simulink model "igct_diode"  (R2023b)
settings: Solver=VariableStepAuto  StartTime=0.0  StopTime=10.0  RelTol=1e-3
values from neighbouring files (symbols this model uses):
  temp_init = 40    [power_sysinit.m]
  Ts1 = 1e-6    (= 1e-06)    [power_sysinit.m]
  Ts2 = 500E-6    (= 0.0005)    [power_sysinit.m]
  Udc = 2500    [power_sysinit.m]
undefined symbols (not defined in the file or in its folder): DIODE_204520, DIODE_344520, DIODE_364520, DIODE_364521, DIODE_D1031SH, DIODE_D1331SH, IGCT_364520_36, IGCT_364521_36, IGCT_654522_6, magnitude, Rch_DIODE, Rch_tau_DIODE, Rjc1_DIODE, Rjc1_tau_DIODE, Rjc2_DIODE, Rjc2_tau_DIODE, Rjc3_DIODE, Rjc3_tau_DIODE, Rth_h, Rth_h_tau
libraries: spsMeanLib x304, simulink x52, spsRMSLib x52
(part 11 of 11)

== system igct_diode/IGCT/36L4521/Subsystem/Subsystem56 ==
  I : Inport
  pwm : Inport  Port=2
  Abs1 : Abs  SaturateOnIntegerOverflow=off
  Add : Sum
  Constant1 : Constant  Value=0
  Constant2 : Constant  Value=0
  Gain1 : Gain  Gain=Udc/IGCT_364521_36.Vdc
  Gain2 : Gain  Gain=IGCT_364521_36.Eon/IGCT_364521_36.IT*Udc/IGCT_364521_36.Vdc
  Gain3 : Gain  Gain=1/Ts2
  Gain4 : Gain
  Logical Operator : Logic  AllPortsSameDT=off  OutDataTypeStr=boolean
  Logical Operator1 : Logic  Operator=NOT  AllPortsSameDT=off  OutDataTypeStr=boolean
  Logical Operator2 : Logic  Operator=NOT  AllPortsSameDT=off  OutDataTypeStr=boolean
  Logical Operator3 : Logic  AllPortsSameDT=off  OutDataTypeStr=boolean
  Logical Operator4 : Logic  AllPortsSameDT=off  OutDataTypeStr=boolean
  Logical Operator5 : Logic  Operator=NOT  AllPortsSameDT=off  OutDataTypeStr=boolean
  Polynomial : Polyval  Coefs=IGCT_364521_36.poly
  Pulse Generator : DiscretePulseGenerator  PulseType=Time based  Period=Ts2  PulseWidth=5
  Switch{1..4} (4 alike) : Switch  Criteria=u2 > Threshold  SaturateOnIntegerOverflow=off  InputSameDT=off
  Unit Delay{,1..3} (4 alike) : UnitDelay  SampleTime=Ts1  HasFrameUpgradeWarning=on
  PS : Outport  VectorParamsAs1DForOutWhenUnconnected=off
  wires:
  pwm/1 -> Logical Operator2/1, Logical Operator/1, Unit Delay/1
  Logical Operator/1 -> Switch1/2
  Abs1/1 -> Add/1
  Switch1/1 -> Abs1/1
  Unit Delay/1 -> Logical Operator3/1, Logical Operator1/1
  Logical Operator1/1 -> Logical Operator/2
  Logical Operator2/1 -> Logical Operator3/2
  Logical Operator3/1 -> Switch2/2
  Constant2/1 -> Switch2/3
  Gain2/1 -> Switch1/1
  Gain1/1 -> Switch1/3
  Switch3/1 -> Add/2
  Constant1/1 -> Switch3/1
  Pulse Generator/1 -> Unit Delay3/1, Logical Operator4/1
  Switch4/1 -> Unit Delay2/1, Gain3/1
  Unit Delay2/1 -> Switch4/3
  Unit Delay3/1 -> Logical Operator5/1
  Logical Operator5/1 -> Logical Operator4/2
  Logical Operator4/1 -> Switch4/2, Switch3/2
  Unit Delay1/1 -> Switch3/3, Switch4/1
  Gain3/1 -> PS/1
  I/1 -> Gain4/1
  Add/1 -> Unit Delay1/1
  Gain4/1 -> Gain2/1, Polynomial/1
  Switch2/1 -> Gain1/1
  Polynomial/1 -> Switch2/1

== system igct_diode/IGCT/36L4521/Subsystem/导通损耗 ==
  note: IGCT导通损耗
  note: 1.39选用的是阈值电压、是否需要改为导通电压
  I : Inport
  Add : Sum
  Gain1 : Gain  Gain=IGCT_364521_36.rT
  Gain2 : Gain  Gain=IGCT_364521_36.VT0
  Gain3 : Gain
  Math Function : Math  Operator=magnitude^2  SignedPower=on
  PD : Outport  VectorParamsAs1DForOutWhenUnconnected=off
  wires:
  Add/1 -> PD/1
  Gain2/1 -> Add/2
  Math Function/1 -> Gain1/1
  I/1 -> Gain3/1
  Gain1/1 -> Add/1
  Gain3/1 -> Gain2/1, Math Function/1

== system igct_diode/IGCT/36L4521/Subsystem/导通损耗1 ==
  note: 1.39选用的是阈值电压、是否需要改为导通电压
  note: IGCT导通损耗
  I : Inport
  Add : Sum
  Gain1 : Gain  Gain=IGCT_364521_36.rT
  Gain2 : Gain  Gain=IGCT_364521_36.VT0
  Gain3 : Gain
  Math Function : Math  Operator=magnitude^2  SignedPower=on
  PD : Outport  VectorParamsAs1DForOutWhenUnconnected=off
  wires:
  Gain3/1 -> Math Function/1, Gain2/1
  Gain1/1 -> Add/1
  I/1 -> Gain3/1
  Math Function/1 -> Gain1/1
  Gain2/1 -> Add/2
  Add/1 -> PD/1

== system igct_diode/IGCT/65L4522/Subsystem/Subsystem1 ==
  I : Inport
  pwm : Inport  Port=2
  Abs1 : Abs  SaturateOnIntegerOverflow=off
  Add : Sum
  Constant1 : Constant  Value=0
  Constant2 : Constant  Value=0
  Gain1 : Gain  Gain=Udc/IGCT_654522_6.Vdc
  Gain2 : Gain  Gain=IGCT_654522_6.Eon/IGCT_654522_6.IT*Udc/IGCT_654522_6.Vdc
  Gain3 : Gain  Gain=1/Ts2
  Gain4 : Gain
  Logical Operator : Logic  AllPortsSameDT=off  OutDataTypeStr=boolean
  Logical Operator1 : Logic  Operator=NOT  AllPortsSameDT=off  OutDataTypeStr=boolean
  Logical Operator2 : Logic  Operator=NOT  AllPortsSameDT=off  OutDataTypeStr=boolean
  Logical Operator3 : Logic  AllPortsSameDT=off  OutDataTypeStr=boolean
  Logical Operator4 : Logic  AllPortsSameDT=off  OutDataTypeStr=boolean
  Logical Operator5 : Logic  Operator=NOT  AllPortsSameDT=off  OutDataTypeStr=boolean
  Polynomial : Polyval  Coefs=IGCT_654522_6.poly
  Pulse Generator : DiscretePulseGenerator  PulseType=Time based  Period=Ts2  PulseWidth=5
  Switch{1..4} (4 alike) : Switch  Criteria=u2 > Threshold  SaturateOnIntegerOverflow=off  InputSameDT=off
  Unit Delay{,1..3} (4 alike) : UnitDelay  SampleTime=Ts1  HasFrameUpgradeWarning=on
  PS : Outport  VectorParamsAs1DForOutWhenUnconnected=off
  wires:
  pwm/1 -> Logical Operator2/1, Logical Operator/1, Unit Delay/1
  Logical Operator/1 -> Switch1/2
  Abs1/1 -> Add/1
  Switch1/1 -> Abs1/1
  Unit Delay/1 -> Logical Operator3/1, Logical Operator1/1
  Logical Operator1/1 -> Logical Operator/2
  Logical Operator2/1 -> Logical Operator3/2
  Logical Operator3/1 -> Switch2/2
  Constant2/1 -> Switch2/3
  Gain2/1 -> Switch1/1
  Gain1/1 -> Switch1/3
  Switch3/1 -> Add/2
  Constant1/1 -> Switch3/1
  Pulse Generator/1 -> Unit Delay3/1, Logical Operator4/1
  Switch4/1 -> Unit Delay2/1, Gain3/1
  Unit Delay2/1 -> Switch4/3
  Unit Delay3/1 -> Logical Operator5/1
  Logical Operator5/1 -> Logical Operator4/2
  Logical Operator4/1 -> Switch4/2, Switch3/2
  Unit Delay1/1 -> Switch3/3, Switch4/1
  Gain3/1 -> PS/1
  I/1 -> Gain4/1
  Add/1 -> Unit Delay1/1
  Gain4/1 -> Gain2/1, Polynomial/1
  Switch2/1 -> Gain1/1
  Polynomial/1 -> Switch2/1

== system igct_diode/IGCT/65L4522/Subsystem/Subsystem2 ==
  note: ch_double
  AVG : Inport
  SW : Inport  Port=2
  Add1 : Sum  Inputs=5
  Add2 : Sum  Inputs=+++
  Add3 : Sum
  Constant1 : Constant  Value=temp_init
  Discrete Filter1 : DiscreteFilter  Numerator=[Ts2/IGCT_654522_6.Rth_ch_dou_tau]  Denominator=[1 (Ts2/IGCT_654522_6.Rth_ch_dou_tau)-1]  SampleTime=Ts2
  Discrete Filter2 : DiscreteFilter  Numerator=[Ts2/IGCT_654522_6.Rth_jc3_dou_tau]  Denominator=[1 (Ts2/IGCT_654522_6.Rth_jc3_dou_tau)-1]  SampleTime=Ts2
  Discrete Filter3 : DiscreteFilter  Numerator=[Ts2/IGCT_654522_6.Rth_jc4_dou_tau]  Denominator=[1 (Ts2/IGCT_654522_6.Rth_jc4_dou_tau)-1]  SampleTime=Ts2
  Discrete Filter5 : DiscreteFilter  Numerator=[Ts2/IGCT_654522_6.Rth_jc1_dou_tau]  Denominator=[1 (Ts2/IGCT_654522_6.Rth_jc1_dou_tau)-1]  SampleTime=Ts2
  Discrete Filter6 : DiscreteFilter  Numerator=[Ts2/IGCT_654522_6.Rth_jc2_dou_tau]  Denominator=[1 (Ts2/IGCT_654522_6.Rth_jc2_dou_tau)-1]  SampleTime=Ts2
  Discrete Filter9 : DiscreteFilter  Numerator=[Ts2/Rth_h_tau]  Denominator=[1 (Ts2/Rth_h_tau)-1]  SampleTime=Ts2
  Gain1 : Gain  Gain=IGCT_654522_6.Rth_ch_dou
  Gain5 : Gain  Gain=IGCT_654522_6.Rth_jc1_dou
  Gain6 : Gain  Gain=IGCT_654522_6.Rth_jc2_dou
  Gain7 : Gain  Gain=IGCT_654522_6.Rth_jc3_dou
  Gain8 : Gain  Gain=IGCT_654522_6.Rth_jc4_dou
  Gain9 : Gain  Gain=Rth_h
  TEMP : Outport  VectorParamsAs1DForOutWhenUnconnected=off
  wires:
  Add3/1 -> Gain9/1, Gain5/1, Gain6/1, Gain7/1, Gain8/1, Gain1/1
  Gain1/1 -> Discrete Filter1/1
  Discrete Filter1/1 -> Add1/5
  Add2/1 -> TEMP/1
  Add1/1 -> Add2/2
  Gain8/1 -> Discrete Filter3/1
  Discrete Filter5/1 -> Add1/1
  Discrete Filter3/1 -> Add1/4
  Discrete Filter2/1 -> Add1/3
  Constant1/1 -> Add2/3
  Gain7/1 -> Discrete Filter2/1
  Discrete Filter6/1 -> Add1/2
  Gain5/1 -> Discrete Filter5/1
  Discrete Filter9/1 -> Add2/1
  Gain9/1 -> Discrete Filter9/1
  Gain6/1 -> Discrete Filter6/1
  SW/1 -> Add3/2
  AVG/1 -> Add3/1

== system igct_diode/IGCT/65L4522/Subsystem/Subsystem31 ==
  note: ch_double
  AVG : Inport
  SW : Inport  Port=2
  Add1 : Sum  Inputs=5
  Add2 : Sum  Inputs=+++
  Add3 : Sum
  Constant1 : Constant  Value=temp_init
  Discrete Filter1 : DiscreteFilter  Numerator=[Ts2/IGCT_654522_6.Rth_ch_dou_tau]  Denominator=[1 (Ts2/IGCT_654522_6.Rth_ch_dou_tau)-1]  SampleTime=Ts2
  Discrete Filter2 : DiscreteFilter  Numerator=[Ts2/IGCT_654522_6.Rth_jc3_dou_tau]  Denominator=[1 (Ts2/IGCT_654522_6.Rth_jc3_dou_tau)-1]  SampleTime=Ts2
  Discrete Filter3 : DiscreteFilter  Numerator=[Ts2/IGCT_654522_6.Rth_jc4_dou_tau]  Denominator=[1 (Ts2/IGCT_654522_6.Rth_jc4_dou_tau)-1]  SampleTime=Ts2
  Discrete Filter5 : DiscreteFilter  Numerator=[Ts2/IGCT_654522_6.Rth_jc1_dou_tau]  Denominator=[1 (Ts2/IGCT_654522_6.Rth_jc1_dou_tau)-1]  SampleTime=Ts2
  Discrete Filter6 : DiscreteFilter  Numerator=[Ts2/IGCT_654522_6.Rth_jc2_dou_tau]  Denominator=[1 (Ts2/IGCT_654522_6.Rth_jc2_dou_tau)-1]  SampleTime=Ts2
  Discrete Filter9 : DiscreteFilter  Numerator=[Ts2/Rth_h_tau]  Denominator=[1 (Ts2/Rth_h_tau)-1]  SampleTime=Ts2
  Gain1 : Gain  Gain=IGCT_654522_6.Rth_ch_dou
  Gain5 : Gain  Gain=IGCT_654522_6.Rth_jc1_dou
  Gain6 : Gain  Gain=IGCT_654522_6.Rth_jc2_dou
  Gain7 : Gain  Gain=IGCT_654522_6.Rth_jc3_dou
  Gain8 : Gain  Gain=IGCT_654522_6.Rth_jc4_dou
  Gain9 : Gain  Gain=Rth_h
  TEMP : Outport  VectorParamsAs1DForOutWhenUnconnected=off
  wires:
  AVG/1 -> Add3/1
  SW/1 -> Add3/2
  Gain6/1 -> Discrete Filter6/1
  Gain9/1 -> Discrete Filter9/1
  Discrete Filter9/1 -> Add2/1
  Gain5/1 -> Discrete Filter5/1
  Discrete Filter6/1 -> Add1/2
  Gain7/1 -> Discrete Filter2/1
  Constant1/1 -> Add2/3
  Discrete Filter2/1 -> Add1/3
  Discrete Filter3/1 -> Add1/4
  Discrete Filter5/1 -> Add1/1
  Gain8/1 -> Discrete Filter3/1
  Add1/1 -> Add2/2
  Add2/1 -> TEMP/1
  Discrete Filter1/1 -> Add1/5
  Gain1/1 -> Discrete Filter1/1
  Add3/1 -> Gain1/1, Gain8/1, Gain7/1, Gain6/1, Gain5/1, Gain9/1

== system igct_diode/IGCT/65L4522/Subsystem/Subsystem56 ==
  I : Inport
  pwm : Inport  Port=2
  Abs1 : Abs  SaturateOnIntegerOverflow=off
  Add : Sum
  Constant1 : Constant  Value=0
  Constant2 : Constant  Value=0
  Gain1 : Gain  Gain=Udc/IGCT_654522_6.Vdc
  Gain2 : Gain  Gain=IGCT_654522_6.Eon/IGCT_654522_6.IT*Udc/IGCT_654522_6.Vdc
  Gain3 : Gain  Gain=1/Ts2
  Gain4 : Gain
  Logical Operator : Logic  AllPortsSameDT=off  OutDataTypeStr=boolean
  Logical Operator1 : Logic  Operator=NOT  AllPortsSameDT=off  OutDataTypeStr=boolean
  Logical Operator2 : Logic  Operator=NOT  AllPortsSameDT=off  OutDataTypeStr=boolean
  Logical Operator3 : Logic  AllPortsSameDT=off  OutDataTypeStr=boolean
  Logical Operator4 : Logic  AllPortsSameDT=off  OutDataTypeStr=boolean
  Logical Operator5 : Logic  Operator=NOT  AllPortsSameDT=off  OutDataTypeStr=boolean
  Polynomial : Polyval  Coefs=IGCT_654522_6.poly
  Pulse Generator : DiscretePulseGenerator  PulseType=Time based  Period=Ts2  PulseWidth=5
  Switch{1..4} (4 alike) : Switch  Criteria=u2 > Threshold  SaturateOnIntegerOverflow=off  InputSameDT=off
  Unit Delay{,1..3} (4 alike) : UnitDelay  SampleTime=Ts1  HasFrameUpgradeWarning=on
  PS : Outport  VectorParamsAs1DForOutWhenUnconnected=off
  wires:
  pwm/1 -> Logical Operator2/1, Logical Operator/1, Unit Delay/1
  Logical Operator/1 -> Switch1/2
  Abs1/1 -> Add/1
  Switch1/1 -> Abs1/1
  Unit Delay/1 -> Logical Operator3/1, Logical Operator1/1
  Logical Operator1/1 -> Logical Operator/2
  Logical Operator2/1 -> Logical Operator3/2
  Logical Operator3/1 -> Switch2/2
  Constant2/1 -> Switch2/3
  Gain2/1 -> Switch1/1
  Gain1/1 -> Switch1/3
  Switch3/1 -> Add/2
  Constant1/1 -> Switch3/1
  Pulse Generator/1 -> Unit Delay3/1, Logical Operator4/1
  Switch4/1 -> Unit Delay2/1, Gain3/1
  Unit Delay2/1 -> Switch4/3
  Unit Delay3/1 -> Logical Operator5/1
  Logical Operator5/1 -> Logical Operator4/2
  Logical Operator4/1 -> Switch4/2, Switch3/2
  Unit Delay1/1 -> Switch3/3, Switch4/1
  Gain3/1 -> PS/1
  I/1 -> Gain4/1
  Add/1 -> Unit Delay1/1
  Gain4/1 -> Gain2/1, Polynomial/1
  Switch2/1 -> Gain1/1
  Polynomial/1 -> Switch2/1

== system igct_diode/IGCT/65L4522/Subsystem/导通损耗 ==
  note: IGCT导通损耗
  note: 1.39选用的是阈值电压、是否需要改为导通电压
  I : Inport
  Add : Sum
  Gain1 : Gain  Gain=IGCT_654522_6.rT
  Gain2 : Gain  Gain=IGCT_654522_6.VT0
  Gain3 : Gain
  Math Function : Math  Operator=magnitude^2  SignedPower=on
  PD : Outport  VectorParamsAs1DForOutWhenUnconnected=off
  wires:
  Add/1 -> PD/1
  Gain2/1 -> Add/2
  Math Function/1 -> Gain1/1
  I/1 -> Gain3/1
  Gain1/1 -> Add/1
  Gain3/1 -> Gain2/1, Math Function/1

== system igct_diode/IGCT/65L4522/Subsystem/导通损耗1 ==
  note: 1.39选用的是阈值电压、是否需要改为导通电压
  note: IGCT导通损耗
  I : Inport
  Add : Sum
  Gain1 : Gain  Gain=IGCT_654522_6.rT
  Gain2 : Gain  Gain=IGCT_654522_6.VT0
  Gain3 : Gain
  Math Function : Math  Operator=magnitude^2  SignedPower=on
  PD : Outport  VectorParamsAs1DForOutWhenUnconnected=off
  wires:
  Gain3/1 -> Math Function/1, Gain2/1
  Gain1/1 -> Add/1
  I/1 -> Gain3/1
  Math Function/1 -> Gain1/1
  Gain2/1 -> Add/2
  Add/1 -> PD/1
